simulink model "n_trotinettes_tout"  (Simulink 6.5)
settings: Solver=ode45  StartTime=0.0  StopTime=L  RelTol=1e-6
undefined symbols (not defined in the file): D, Delta, dt, gama, Imax, Ka, Ki, KphiSJv, Kpwm, Ktach, Kv, M_ecart, N, NDelta, NKtach, Si, start, stop
settings Model: Creator=admin  LastModifiedBy=admin
settings DataIOCC: SignalLoggingName=sigsOut
settings DebuggingCC: SolverPrmCheckMsg=none  MultiTaskDSMMsg=warning  MultiTaskCondExecSysMsg=none  StrictBusMsg=None
settings HardwareCC: TargetUnknown=on
settings RTWCC: IncludeERTFirstTime=on

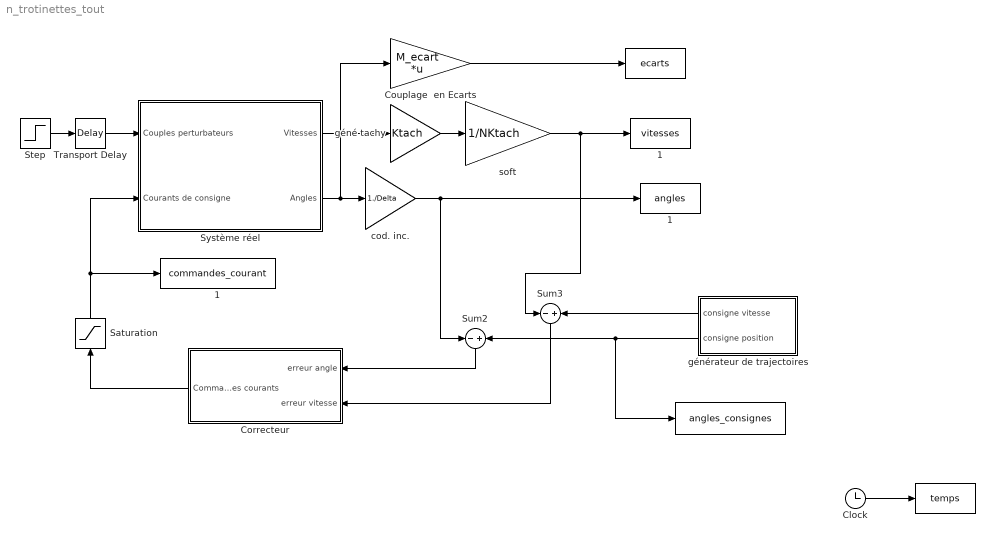
== system n_trotinettes_tout ==
  " " : ToWorkspace  VariableName=temps  SampleTime=-1  SaveFormat=Array
  "  " : ToWorkspace  VariableName=angles_consignes  SampleTime=-1  SaveFormat=Array
  "   " : ToWorkspace  VariableName=ecarts  SampleTime=-1  SaveFormat=Array
  "  1" : ToWorkspace  VariableName=angles  SampleTime=-1  SaveFormat=Array
  " 1" : ToWorkspace  VariableName=vitesses  SampleTime=-1  SaveFormat=Array
  "   1" : ToWorkspace  VariableName=commandes_courant  SampleTime=-1  SaveFormat=Array
  Clock : Clock
      settings: Decimation=10
  Correcteur : Subsystem  Orientation=left
  Couplage  en Ecarts : Gain  Gain=M_ecart  Multiplication=Matrix(K*u)  SaturateOnIntegerOverflow=on
  Saturation : Saturate  Orientation=up  UpperLimit=+Imax  LowerLimit=-Imax
  Step : Step  Time=(start+stop)/2  Before=zeros(N,1)  After=ones(N,1)*4  SampleTime=0
  Sum2 : Sum  Orientation=down  Inputs=-|+  SaturateOnIntegerOverflow=on
  Sum3 : Sum  Orientation=down  Inputs=-|+  SaturateOnIntegerOverflow=on
  Système réel : Subsystem
  Transport Delay : TransportDelay  DelayTime=0:0.3:(N-1)*0.3  InitialOutput=zeros(N,1)
  cod. inc. : Gain  Gain=1./Delta  SaturateOnIntegerOverflow=on
  géné tachy : Gain  Gain=Ktach  SaturateOnIntegerOverflow=on
  générateur de trajectoires : Subsystem  Orientation=left
  soft : Gain  Gain=1/NKtach  SaturateOnIntegerOverflow=on
  wires:
  Système réel/2(Angles) -> cod. inc./1, Couplage  en Ecarts/1
  générateur de trajectoires/2(consigne position) -> Sum2/2, "  "/1
  Clock/1 -> " "/1
  Correcteur/1(Commandes courants) -> Saturation/1
  Système réel/1(Vitesses) -> géné tachy/1
  Sum3/1 -> Correcteur/2(erreur vitesse)
  Sum2/1 -> Correcteur/1(erreur angle)
  générateur de trajectoires/1(consigne vitesse) -> Sum3/2
  Couplage  en Ecarts/1 -> "   "/1
  géné tachy/1 -> soft/1
  cod. inc./1 -> Sum2/1, "  1"/1
  Saturation/1 -> Système réel/2(Courants de consigne), "   1"/1
  soft/1 -> Sum3/1, " 1"/1
  Step/1 -> Transport Delay/1
  Transport Delay/1 -> Système réel/1(Couples perturbateurs)

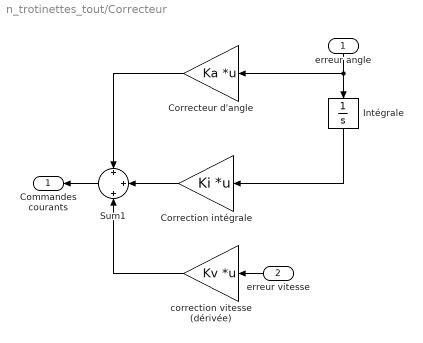
== system n_trotinettes_tout/Correcteur ==
  erreur angle : Inport  Orientation=down
  erreur vitesse : Inport  Orientation=left  Port=2
  Correcteur d'angle : Gain  Orientation=left  Gain=Ka  Multiplication=Matrix(K*u)  SaturateOnIntegerOverflow=on
  Correction intégrale : Gain  Orientation=left  Gain=Ki  Multiplication=Matrix(K*u)  SaturateOnIntegerOverflow=on
  Intégrale : Integrator  Orientation=down  InitialCondition=zeros(N,1)
  Sum1 : Sum  Orientation=left  Inputs=+|+|+  SaturateOnIntegerOverflow=on  InputSameDT=on
  correction vitesse (dérivée) : Gain  Orientation=left  Gain=Kv  Multiplication=Matrix(K*u)  SaturateOnIntegerOverflow=on
  Commandes courants : Outport  Orientation=left
  wires:
  erreur angle/1 -> Correcteur d'angle/1, Intégrale/1
  Correcteur d'angle/1 -> Sum1/1
  Intégrale/1 -> Correction intégrale/1
  correction vitesse (dérivée)/1 -> Sum1/3
  Correction intégrale/1 -> Sum1/2
  Sum1/1 -> Commandes courants/1
  erreur vitesse/1 -> correction vitesse (dérivée)/1

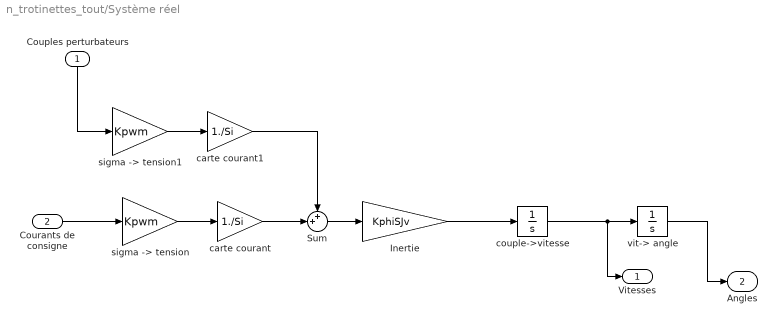
== system n_trotinettes_tout/Système réel ==
  Couples perturbateurs : Inport  Orientation=down
  Courants de consigne : Inport  Port=2
  Inertie : Gain  Gain=KphiSJv  SaturateOnIntegerOverflow=on
  Sum : Sum  Inputs=++|  SaturateOnIntegerOverflow=on
  carte courant : Gain  Gain=1./Si  SaturateOnIntegerOverflow=on
  carte courant1 : Gain  Gain=1./Si  SaturateOnIntegerOverflow=on
  couple->vitesse : Integrator  InitialCondition=zeros(N,1)
  "sigma -> tension" : Gain  Gain=Kpwm  SaturateOnIntegerOverflow=on
  "sigma -> tension1" : Gain  Gain=Kpwm  SaturateOnIntegerOverflow=on
  vit-> angle : Integrator  InitialCondition=(0:N-1)*D
  Vitesses : Outport
  Angles : Outport  Port=2
  wires:
  couple->vitesse/1 -> vit-> angle/1, Vitesses/1
  carte courant/1 -> Sum/2
  Sum/1 -> Inertie/1
  vit-> angle/1 -> Angles/1
  Courants de consigne/1 -> "sigma -> tension"/1
  "sigma -> tension"/1 -> carte courant/1
  Inertie/1 -> couple->vitesse/1
  Couples perturbateurs/1 -> "sigma -> tension1"/1
  "sigma -> tension1"/1 -> carte courant1/1
  carte courant1/1 -> Sum/1

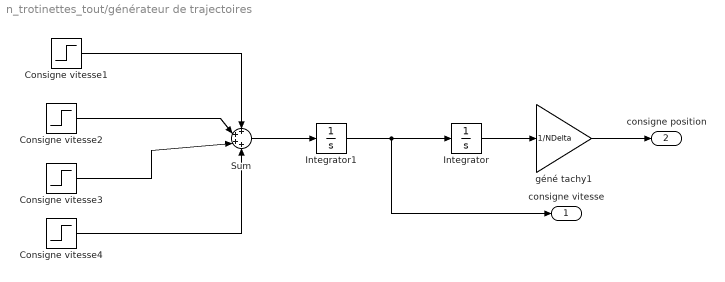
== system n_trotinettes_tout/générateur de trajectoires ==
  Consigne vitesse1 : Step  Time=start  After=gama  SampleTime=0
  Consigne vitesse2 : Step  Time=start+dt  After=-gama  SampleTime=0
  Consigne vitesse3 : Step  Time=stop  After=-gama  SampleTime=0
  Consigne vitesse4 : Step  Time=stop+dt  After=gama  SampleTime=0
  Integrator : Integrator  InitialCondition=(0:N-1)'*D
  Integrator1 : Integrator  InitialCondition=zeros(N,1)
  Sum : Sum  Inputs=++++
  géné tachy1 : Gain  Gain=1/NDelta  SaturateOnIntegerOverflow=on
  consigne vitesse : Outport
  consigne position : Outport  Port=2
  wires:
  Integrator1/1 -> Integrator/1, consigne vitesse/1
  Integrator/1 -> géné tachy1/1
  géné tachy1/1 -> consigne position/1
  Consigne vitesse1/1 -> Sum/1
  Consigne vitesse2/1 -> Sum/2
  Consigne vitesse3/1 -> Sum/3
  Consigne vitesse4/1 -> Sum/4
  Sum/1 -> Integrator1/1
